simulink model "WT_test1"  (R2022a)
settings: Solver=VariableStepAuto  StartTime=0.0  StopTime=10  RelTol=1e-3
settings Model: Creator=smiu  LastModifiedBy=smiu
settings DataIOCC: ExternalInput=[Fy]
settings DebuggingCC: UnconnectedInputMsg=warning  UnconnectedOutputMsg=warning  UnconnectedLineMsg=warning
settings RTWCC: DLArmComputeVersion=19.05

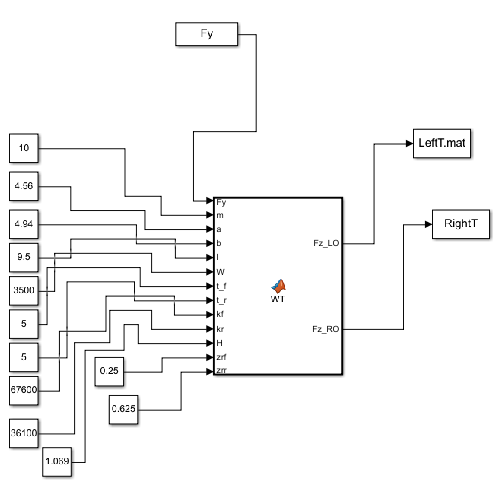
[thumbnail: Simulink's stored preview of the top-level diagram]
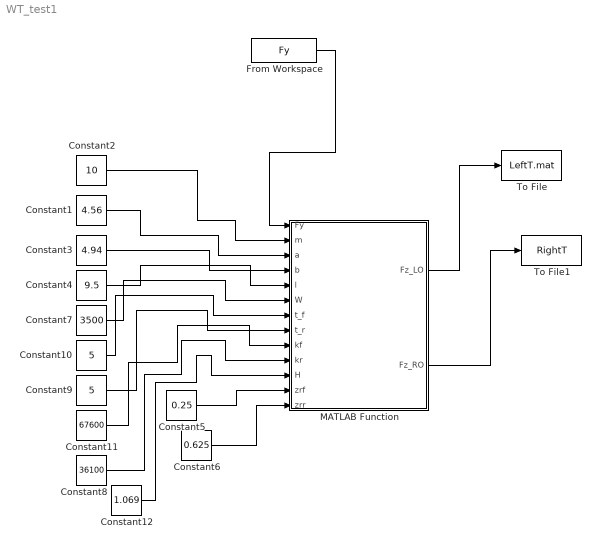
== system WT_test1 ==
  Constant1 : Constant  Value=4.56
  Constant10 : Constant  Value=5
  Constant11 : Constant  Value=67600
  Constant12 : Constant  Value=1.069
  Constant2 : Constant  Value=10
  Constant3 : Constant  Value=4.94
  Constant4 : Constant  Value=9.5
  Constant5 : Constant  Value=0.25
  Constant6 : Constant  Value=0.625
  Constant7 : Constant  Value=3500
  Constant8 : Constant  Value=36100
  Constant9 : Constant  Value=5
  From Workspace : FromWorkspace  VariableName=Fy  OutDataTypeStr=double
  MATLAB Function : MATLAB Function  TreatAsAtomicUnit=on
  To File : ToFile  Filename=LeftT.mat  MatrixName=FzL  SaveFormat=Timeseries
  To File1 : ToFile  Filename=RightT  MatrixName=FzR  SaveFormat=Timeseries
  wires:
  Constant1/1 -> MATLAB Function/3(a)
  Constant2/1 -> MATLAB Function/2(m)
  From Workspace/1 -> MATLAB Function/1(Fy)
  Constant6/1 -> MATLAB Function/13(zrr)
  Constant5/1 -> MATLAB Function/12(zrf)
  Constant3/1 -> MATLAB Function/4(b)
  Constant4/1 -> MATLAB Function/5(l)
  Constant7/1 -> MATLAB Function/6(W)
  Constant10/1 -> MATLAB Function/7(t_f)
  Constant9/1 -> MATLAB Function/8(t_r)
  Constant11/1 -> MATLAB Function/9(kf)
  Constant8/1 -> MATLAB Function/10(kr)
  Constant12/1 -> MATLAB Function/11(H)
  MATLAB Function/1(Fz_LO) -> To File/1
  MATLAB Function/2(Fz_RO) -> To File1/1

== matlab function WT_test1/MATLAB Function ==
  data: Fy input; Fz_LO output; m input; a input; Fz_RO output; b input; l input; W input; t_f input; t_r input; kf input; kr input; H input; zrf input; zrr input
function [Fz_LO,Fz_RO] = WT(Fy,m,a,b,l,W,t_f,t_r,kf,kr,H,zrf,zrr)
%for i=1:length(Fy)
 %   if Fy(i) < 0
  %      Fy(i) = abs(Fy(i));
   % end
%end
%A_x = Fx/m;
A_y = Fy/m;
W_F = W * b/l;
%value check for negitive input
W_R = W * a/l;
delta_F = A_y * (W/t_f)*((H*kf)/(kf+kr) + (b/l) * zrf);
delta_R = A_y * (W/t_r)*((H*kr)/(kf+kr) + (a/l) * zrr);
W_Fo = (W_F/2) + (delta_F); 
W_Fi = (W_F/2) - (delta_F);
W_Ro = (W_R/2) + (delta_R);
W_Ri = (W_R/2) - (delta_R);
Fz_LO = [W_Fo,W_Fi];
Fz_RO = [W_Ro,W_Ri];
end
